simulink model "faulttest"  (R2023b)
settings: Solver=ode4  StartTime=0.0  StopTime=5  FixedStep=0.0005  RelTol=1e-3  AbsTol=1e-6
libraries: eeRmsMeasurement x8, spsSeriesRLCBranchLib x3, spsAsynchronousMachineSIUnitsLib x1, eePowerMeasurement x1, spsThreePhaseVIMeasurementLib x1, spsThreePhaseSourceLib x1, spspowerguiLib x1
settings Model: SimulationMode=accelerator  Creator=edemk  LastModifiedBy=edemk

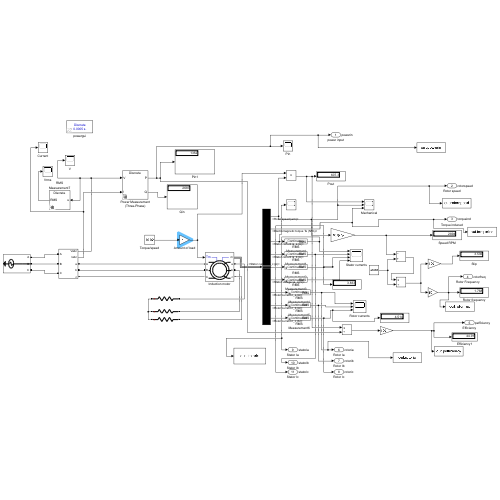
[thumbnail: Simulink's stored preview of the top-level diagram]
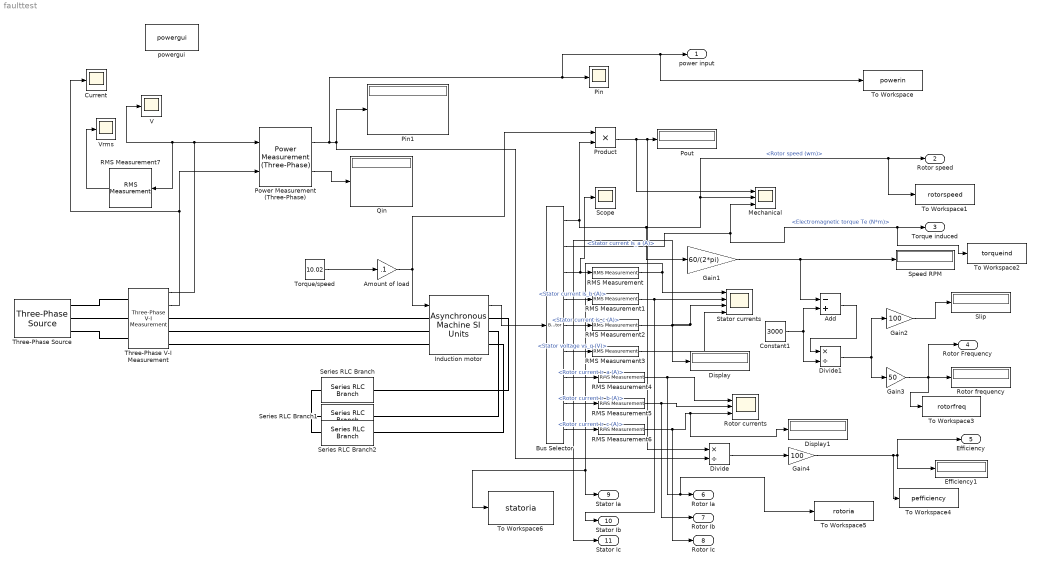
== system faulttest ==
  Add : Sum  Inputs=-+
  Amount of load : Gain  Gain=.1
  Bus Selector : BusSelector  OutputSignals=Mechanical.Rotor speed (wm),Mechanical.Electromagnetic torque Te (N*m),Stator measurements.Stator current is_a (A),Stator measurements.Stator current is_b (A),Stator measurements.Stator current is_c (A),Stator measurements.Stator voltage vs_q (V),Rotor measurements.Rotor current ir_a (A),Rotor measurements.Rotor current ir_b (A),Rotor measurements.Rotor current ir_c (A)
  Constant1 : Constant  Value=3000
  Current : Scope
  Display : Display
  Display1 : Display
  Divide : Product  Inputs=*/
  Divide1 : Product  Inputs=*/
  Efficiency1 : Display
  Gain1 : Gain  Gain=60/(2*pi)
  Gain2 : Gain  Gain=100
  Gain3 : Gain  Gain=50
  Gain4 : Gain  Gain=100
  Induction motor : spsAsynchronousMachineSIUnitsLib/Asynchronous Machine SI Units  RotorType=Wound  PresetModel=No  MechanicalLoad=Torque Tm  ShowDetailedParameters=on  ReferenceFrame=Rotor  Units=SI  MeasurementBus=off  NominalParameters=[3000 415 50]  VoltageRatio=0.5  Stator=[4.989 0.0002408]  Rotor=[1.1 0.006]  Cage1=[3.764 0.002454]  Cage2=[3.784 0.002408]  Lm=0.1907  Mechanical=[0.02 0.005 1]  PolePairs=2  InitialConditions=[0 0 0 0 0 0 0 0]  SimulateSaturation=off  Saturation=[14.03593122, 27.81365428, 53.79336849, 72.68890987, 97.98006896, 148.6815601, 215.7428561, 302.9841135, 428.7778367 ; 230, 322, 414, 460, 506, 552, 598, 644, 690]  LoadFlowParameters=1492000  TsPowergui=0  TsBlock=-1  IterativeModel=Trapezoidal non iterative  IterativeDiscreteModel=Trapezoidal non iterative  Pmec=3000
  Mechanical : Scope  NumInputPorts=3
  Pin : Scope
  Pin1 : Display
  Pout : Display
  Power Measurement (Three-Phase) : eePowerMeasurement/Power Measurement (Three-Phase)  LabelModeActiveChoice=Discrete  F=50  K=[1]  Seq=Positive  Ts=0.0005
  Product : Product
  Qin : Display
  RMS Measurement{,1..6} (7 alike) : eeRmsMeasurement/RMS Measurement  LabelModeActiveChoice=Total  F=60  SpecifyHarmonics=off  K=[0 1 2]  Ts=0
      settings: LibrarySourceBlock=|
      | ee_sl_lib/Measurements/RMS
      | Measurement
  RMS Measurement7 : eeRmsMeasurement/RMS Measurement  LabelModeActiveChoice=Total  F=50  SpecifyHarmonics=off  K=[0 1 2]  Ts=0.0005
      settings: LibrarySourceBlock=|
      | ee_sl_lib/Measurements/RMS
      | Measurement
  Rotor currents : Scope  NumInputPorts=3
  Rotor frequency : Display
  Scope : Scope
  Series RLC Branch : spsSeriesRLCBranchLib/Series RLC Branch  LConnTagsString=__new0  RConnTagsString=__new0  BranchType=R  Resistance=1  Inductance=1e-3  SetiL0=off  InitialCurrent=0  Capacitance=1e-6  Setx0=off  InitialVoltage=0  Measurements=None
  Series RLC Branch1 : spsSeriesRLCBranchLib/Series RLC Branch  LConnTagsString=__new0  RConnTagsString=__new0  BranchType=R  Resistance=1  Inductance=1e-3  SetiL0=off  InitialCurrent=0  Capacitance=1e-6  Setx0=off  InitialVoltage=0  Measurements=None
  Series RLC Branch2 : spsSeriesRLCBranchLib/Series RLC Branch  LConnTagsString=__new0  RConnTagsString=__new0  BranchType=R  Resistance=1  Inductance=1e-3  SetiL0=off  InitialCurrent=0  Capacitance=1e-6  Setx0=off  InitialVoltage=0  Measurements=None
  Slip : Display
  Speed RPM : Display
  Stator currents : Scope  NumInputPorts=4
  Three-Phase V-I Measurement : spsThreePhaseVIMeasurementLib/Three-Phase V-I Measurement  VoltageMeasurement=phase-to-ground  SetLabelV=off  LabelV=Vabc  Vpu=off  VpuLL=off  CurrentMeasurement=yes  SetLabelI=off  LabelI=Iabc  Ipu=off  Pbase=100e6  Vbase=500e3  OutputType=Complex  PhasorSimulation=off  PSBequivalent=0
  Three-Phase Source : spsThreePhaseSourceLib/Three-Phase Source  InternalConnection=Yg  VoltagePhases=off  Voltage=415  PhaseAngle=0  Voltage_phases=[ 230.94 230.94 230.94]/sqrt(3)  PhaseAngles_phases=[0 +120 -120]  Frequency=50  NonIdealSource=on  SpecifyImpedance=off  Resistance=0  Inductance=0  ShortCircuitLevel=100e6  BaseVoltage=0  XRratio=7  BusType=swing  Pref=10e3  Qref=0  Prefabc=[10e3, 10e3, 10e3]  Qrefabc=[0, 0, 0]  Qmin=-inf  Qmax=inf
  To Workspace : ToWorkspace  VariableName=powerin  SampleTime=-1
  To Workspace1 : ToWorkspace  VariableName=rotorspeed  SampleTime=-1
  To Workspace2 : ToWorkspace  VariableName=torqueind  SampleTime=-1
  To Workspace3 : ToWorkspace  VariableName=rotorfreq  SampleTime=-1
  To Workspace4 : ToWorkspace  VariableName=pefficiency  SampleTime=-1
  To Workspace5 : ToWorkspace  VariableName=rotoria  SampleTime=-1
  To Workspace6 : ToWorkspace  VariableName=statoria  SampleTime=-1
  Torque/speed : Constant  Value=10.02  SampleTime=0.0005
  V : Scope
  Vrms : Scope
  powergui : spspowerguiLib/powergui  Priority=1  SimulationMode=Discrete  SampleTime=5e-4  frequency=60  Iterations=50  frequencyindice=50  Pbase=100e6  ErrMax=1e-4  UnitsV=kV  UnitsW=MW  buscounter=0  FunctionMessages=off  echomessages=off  EnableUseOfTLC=off  CurrentSourceSwitches=off  DisableSnubberDevices=off  DisableRonSwitches=off  DisableVfSwitches=off  DisplayEquations=off  AutomaticDiscreteSolvers=off  SolverType=Tustin/Backward Euler (TBE)  Interpol=off  ExternalGateDelay=off  methode=off  Ts=100  x0status=blocks  SPID=on  SwTol=0  HookPort=off  NonlinearTolerance=1e-4  nMaxIteration=100  ContinueOnMaxIteration=off  RestoreLinks=warning  ResistiveCurrentMeasurement=off  Frange=[0:2:500]  Ylog=off  Xlog=on  ShowGrid=off  save=off  variable=ZData  structure=0  ZoomFFT=off  StartTime=0.0  cycles=1  DisplayStyle=1  fundamental=60  FreqAxis=off  MaxFrequency=1000  frequencyindicesteady=1  RmsSteady=1  display=off
  power input : Outport  SignalName=powerin
  Rotor speed : Outport  Port=2  SignalName=rotorspeed
  Torque induced : Outport  Port=3  SignalName=torqueind
  Rotor Frequency : Outport  Port=4  SignalName=rotorfreq
  Efficiency : Outport  Port=5  SignalName=pefficiency
  Rotor Ia : Outport  Port=6  SignalName=rotoria
  Rotor Ib : Outport  Port=7  SignalName=rotorib
  Rotor Ic : Outport  Port=8  SignalName=rotoric
  Stator Ia : Outport  Port=9  SignalName=statoria
  Stator Ib : Outport  Port=10  SignalName=statorib
  Stator Ic : Outport  Port=11  SignalName=statoric
  wires:
  Three-Phase V-I Measurement/1 -> RMS Measurement7/1, V/1, Power Measurement (Three-Phase)/1
  Three-Phase V-I Measurement/2 -> Power Measurement (Three-Phase)/2, Current/1
  Induction motor/1 -> Bus Selector/1
  Power Measurement (Three-Phase)/2 -> Qin/1
  Power Measurement (Three-Phase)/1 -> Divide/2, Pin1/1, To Workspace/1, power input/1, Pin/1
  Amount of load/1 -> Induction motor/1, Product/1
  Bus Selector/1 -> Product/2, Gain1/1, To Workspace1/1, Rotor speed/1, Mechanical/2  "<Rotor speed (wm)>"
  Product/1 -> Divide/1, Pout/1, Mechanical/1
  Bus Selector/2 -> To Workspace2/1, Torque induced/1, Mechanical/3  "<Electromagnetic torque Te (N*m)>"
  Gain1/1 -> Add/1, Speed RPM/1
  Bus Selector/3 -> Scope/1, RMS Measurement/1  "<Stator current is_a (A)>"
  RMS Measurement/1 -> To Workspace6/1, Stator Ia/1, Stator currents/1
  RMS Measurement1/1 -> Stator currents/2, Stator Ib/1
  Bus Selector/4 -> RMS Measurement1/1  "<Stator current is_b (A)>"
  Bus Selector/5 -> RMS Measurement2/1  "<Stator current is_c (A)>"
  RMS Measurement2/1 -> Stator Ic/1, Stator currents/3, Display/1
  Bus Selector/6 -> RMS Measurement3/1  "<Stator voltage vs_q (V)>"
  RMS Measurement3/1 -> Stator currents/4
  RMS Measurement5/1 -> Rotor Ib/1, Rotor currents/2
  RMS Measurement4/1 -> To Workspace5/1, Rotor Ia/1, Rotor currents/1
  Bus Selector/7 -> RMS Measurement4/1  "<Rotor current ir_a (A)>"
  Bus Selector/8 -> RMS Measurement5/1  "<Rotor current ir_b (A)>"
  Bus Selector/9 -> RMS Measurement6/1  "<Rotor current ir_c (A)>"
  Constant1/1 -> Divide1/2, Add/2
  Add/1 -> Divide1/1
  Gain2/1 -> Slip/1
  Divide1/1 -> Gain2/1, Gain3/1
  Gain3/1 -> Rotor Frequency/1, To Workspace3/1, Rotor frequency/1
  Gain4/1 -> Efficiency/1, Efficiency1/1, To Workspace4/1
  Divide/1 -> Gain4/1
  RMS Measurement7/1 -> Vrms/1
  RMS Measurement6/1 -> Rotor Ic/1, Display1/1, Rotor currents/3
  Torque/speed/1 -> Amount of load/1
  connections:
  Three-Phase Source/RConn2 -- Three-Phase V-I Measurement/LConn2
  Three-Phase V-I Measurement/LConn1 -- Three-Phase Source/RConn1
  Three-Phase V-I Measurement/LConn3 -- Three-Phase Source/RConn3
  Three-Phase V-I Measurement/RConn2 -- Induction motor/LConn2
  Three-Phase V-I Measurement/RConn3 -- Induction motor/LConn3
  Induction motor/LConn1 -- Three-Phase V-I Measurement/RConn1
  Series RLC Branch/LConn1 -- Series RLC Branch2/LConn1 -- Series RLC Branch1/LConn1
  Induction motor/RConn1 -- Series RLC Branch/RConn1
  Induction motor/RConn2 -- Series RLC Branch1/RConn1
  Induction motor/RConn3 -- Series RLC Branch2/RConn1
